simulink model "PID"  (R2019a)
settings: Solver=VariableStepAuto  StartTime=0.0  StopTime=10  RelTol=1e-5
settings Model: Creator=AS  LastModifiedBy=AS

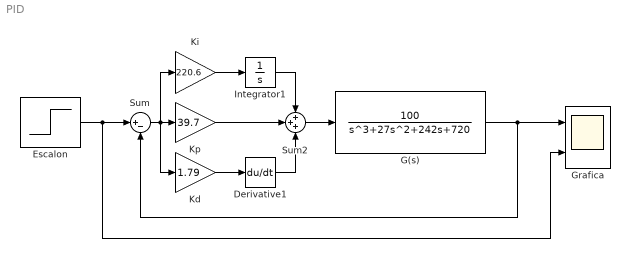
== system PID ==
  Derivative1 : Derivative
  "Escalon " : Step  SampleTime=0
  "G(s) " : TransferFcn  Numerator=[100]  Denominator=[1,27,242,720]
  "Grafica " : Scope  NumInputPorts=2
  Integrator1 : Integrator
  Kd : Gain  Gain=1.79
  Ki : Gain  Gain=220.6
  Kp : Gain  Gain=39.7
  Sum : Sum  Inputs=|+-
  Sum2 : Sum  Inputs=+++
  wires:
  "G(s) "/1 -> Sum/2, "Grafica "/1
  "Escalon "/1 -> "Grafica "/2, Sum/1
  Kd/1 -> Derivative1/1
  Ki/1 -> Integrator1/1
  Integrator1/1 -> Sum2/1
  Kp/1 -> Sum2/2
  Derivative1/1 -> Sum2/3
  Sum2/1 -> "G(s) "/1
  Sum/1 -> Kd/1, Ki/1, Kp/1
